simulink model "Lab_1_sim"  (R2017a)
settings: Solver=VariableStepAuto  StartTime=0.0  StopTime=1.0  RelTol=1e-3
values from neighbouring files (symbols this model uses):
  alpha = 26.66667    [Lab_1.m]
  beta = 133.33333    [Lab_1.m]
  K = f*(alpha_p.^2)/(4*beta)    [Lab_1.m]
undefined symbols (not defined in the file or in its folder): c1, c2
settings Model: Creator=njohnson  LastModifiedBy=njohnson

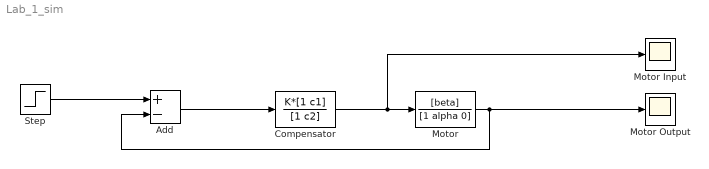
== system Lab_1_sim ==
  Add : Sum  Inputs=+-
  "Compensator " : TransferFcn  Numerator=K*[1 c1]  Denominator=[1 c2]
  "Motor " : TransferFcn  Numerator=[beta]  Denominator=[1 alpha 0]
  Motor Input : Scope
  Motor Output : Scope
  Step : Step  Time=0  After=3  SampleTime=0
  wires:
  Step/1 -> Add/1
  Add/1 -> "Compensator "/1
  "Compensator "/1 -> Motor Input/1, "Motor "/1
  "Motor "/1 -> Motor Output/1, Add/2
